simulink model "ten"  (R2020b)
settings: Solver=VariableStepAuto  StartTime=0.0  StopTime=10.0  RelTol=1e-3
values from neighbouring files (symbols this model uses):
  Kd = 1    [Control_lab2_ex10.m]    (also in Control_lab2_ex10_2.m = 0)
  Ki = 1    [Control_lab2_ex10.m]    (also in Control_lab2_ex10_2.m = 0)
  Kp = 1    [Control_lab2_ex10.m]    (also in Control_lab2_ex10_2.m; Control_lab2_ex2.m = 140; Control_lab2_ex3b.m = 100; Control_lab2_ex4.m = 100)
settings Model: Creator=20775  LastModifiedBy=20775

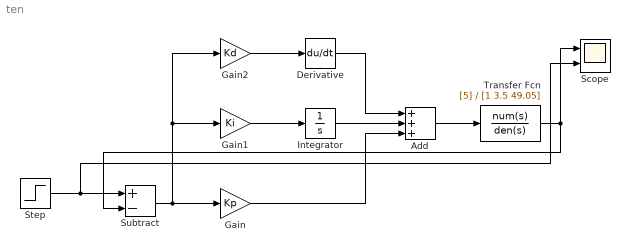
== system ten ==
  Add : Sum  Inputs=+++
  Derivative : Derivative
  Gain : Gain  Gain=Kp
  Gain1 : Gain  Gain=Ki
  Gain2 : Gain  Gain=Kd
  Integrator : Integrator
  Scope : Scope  NumInputPorts=2
  Step : Step  SampleTime=0
  Subtract : Sum  Inputs=+-
  Transfer Fcn : TransferFcn  Numerator=[5]  Denominator=[1 3.5 49.05]
  wires:
  Step/1 -> Scope/2, Subtract/1
  Subtract/1 -> Gain2/1, Gain1/1, Gain/1
  Gain2/1 -> Derivative/1
  Gain1/1 -> Integrator/1
  Gain/1 -> Add/3
  Integrator/1 -> Add/2
  Derivative/1 -> Add/1
  Add/1 -> Transfer Fcn/1
  Transfer Fcn/1 -> Scope/1, Subtract/2
